simulink library "sm_suspension_templates_lib"  (R2021b)
settings: Solver=ode45  StartTime=0.0  StopTime=10.0  RelTol=1e-3  EnableMultiTasking=on
undefined symbols (not defined in the file or in its folder): dgrey, lbrown, lgrey, orange, rho_alum, X, Y, Z
libraries: sm_lib x133, $bdroot x10, nesl_utility x3, sm_double_wishbone_suspension_lib x2
(part 1 of 4)
settings Model: Creator=The MathWorks, Inc.  LastModifiedBy=The MathWorks, Inc.
settings SolverCC: AlgebraicLoopSolver=TrustRegion
settings DataIOCC: LimitDataPoints=on  SaveFormat=Array  ReturnWorkspaceOutputs=off
settings OptimizationCC: ExpressionDepthLimit=2147483647  LifeSpan=inf
settings DebuggingCC: UnderspecifiedInitializationDetection=Classic  MergeDetectMultiDrivingBlocksExec=none  SolverPrmCheckMsg=warning  AllowSymbolicDim=off  StateNameClashWarn=warning  SFUnexpectedBacktrackingDiag=warning  SFNoUnconditionalDefaultTransitionDiag=warning  SFExecutionAtInitializationDiag=none  SFMachineParentedDataDiag=warning  ArithmeticOperatorsInVariantConditions=warning
settings HardwareCC: ProdBitPerPointer=32  ProdBitPerSizeT=32  ProdBitPerPtrDiffT=32  ProdLargestAtomicFloat=None  ProdIntDivRoundTo=Undefined  ProdEndianess=Unspecified  ProdWordSize=32  ProdHWDeviceType=32-bit Generic
settings ModelReferenceCC: PropagateSignalLabelsOutOfModel=off
settings SFSimCC: SimUseLocalCustomCode=off  CustomCodeUndefinedFunction=UseInterfaceOnly
settings RTWCC: RTWUseLocalCustomCode=off
settings CodeAppCC: StateflowObjectComments=on
settings GRTTargetCC: TargetLangStandard=C89/C90 (ANSI)
settings ConfigComp: CovMetricSettings=dw  CovSaveCumulativeToWorkspaceVar=on  CovSaveSingleToWorkspaceVar=on  CovExternalEMLEnable=off  CovSFcnEnable=off

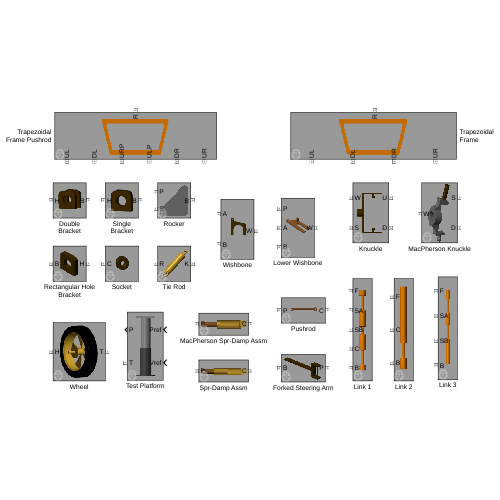
[thumbnail: Simulink's stored preview of the top-level diagram]
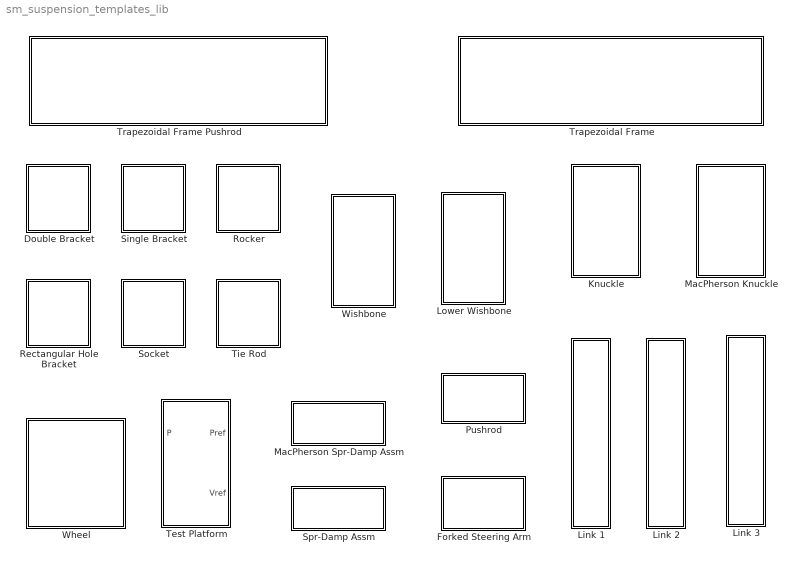
== system sm_suspension_templates_lib ==
  Double Bracket : Subsystem  mask(Bracket){L=4, W=4, T=1, S=1.5, Rh=1, rho=2700, clr=[0.3 0.2 0]}
      mask prompts: L "Length (cm):"; W "Width (cm):"; T "Thickness (cm):"; S "Spacing (cm):"; Rh "Hole radius (cm):"; rho "Density (kg/m^3):"; clr "Color ([r g b]):"
      mask help: This block models a rectangular bracket with two flanges. The port B corresponds to the base of the bracket and the port H corresponds to the bracket hole.
      mask init:
      | bracket_xsec = [W/2 -L/2; W/2 L/2; -W/2 L/2; -W/2 -L/2];
      | bracket_xsec = simmechanics.demohelpers.round_corners(bracket_xsec,[2 3],1,5);
      | 
      | theta = linspace(3*pi/2,-pi/2,100)';
      | bracket_xsec = [bracket_xsec; bracket_xsec(1,:);
      |                 Rh*cos(theta) Rh*sin(theta)];
      mask DialogControl ParameterTabVar0 Prompt: Dimensions
      mask DialogControl ParameterTabVar01 Prompt: Material Properties
      mask Display:
      | image(imread(fullfile(matlabroot,...
      |     'toolbox','physmod','sm','smdemos',...
      |     'suspension_templates','images','sm_isuspension_dbracket.png')));
      | 
      | port_label('LConn',1,'H');
      | port_label('RConn',1,'B');
  Forked Steering Arm : Subsystem  mask(Forked Steering Arm){L=20, W=2, Lf=4, Hf=10, Of=0, T=1, Rp=0.25, Rr=0.25, rho=2700, clr=[0.3 0.2 0]}
      mask prompts: L "Length of link (cm):"; W "Width of link (cm):"; Lf "Length of forked section (cm):"; Hf "Height of forked section (cm):"; Of "Offset of forked section (cm):"; T "Thickness of link (cm):"; Rp "Pin radius (cm):"; Rr "Chamfer/fillet radius (cm):"; rho "Density (kg/m^3)"; clr "Color ([r g b]):"
      mask help: This block models a steering arm that rigidly connects to the steering knuckle and is pushed/pulled by the tie rod to steer the vehicle. The port B corresponds to the attachment point of the arm to the knuckle and the port P refers to the pin frame where the arm attaches to the tie rod.
      mask init:
      | fork_xsec = [ -(L-Lf+T/2) -T/2; 
      |               -T/2 -T/2; 
      |               -T/2 -Hf/2+Of;
      |               Lf-T/2 -Hf/2+Of; 
      |               Lf-T/2 -(Hf/2-T)+Of; 
      |               T/2 -(Hf/2-T)+Of;
      |               T/2 (Hf/2-T)+Of; 
      |               Lf-T/2 (Hf/2-T)+Of; 
      |               Lf-T/2 Hf/2+Of;
      |               -T/2 Hf/2+Of;  
      |               -T/2 T/2; 
      |               -(L-Lf+T/2) T/2];
      | 
      | fork_xsec = simmechanics.demohelpers.round_corners(fork_xsec,2:11,Rr,5);
      mask DialogControl ParameterTabVar0 Prompt: Dimensions
      mask DialogControl ParameterTabVar01 Prompt: Material Properties
      mask Display:
      | image(fullfile(matlabroot,'toolbox','physmod','sm','smdemos','suspension_templates','images','sm_isuspension_steerarm.png'));
      | port_label('LConn',1,'B');
      | port_label('RConn',1,'P');
  Knuckle : Subsystem  mask(Steering knuckle){H=43, L=8, T=1, Wpr=2.5, Hpr=8, Wc=10, Rd=2, Hd=6, Rr=0.3, Rt=2, Rb=1, Rp=0.5, Hp=3, Ls=20, Ws=2, Ts=1, Hsf=10, Lsf=4, Osf=0, Rsp=0.5, Rsr=0.25, Rev=off, rho=2700, clr=[0.5 0.5 0.5]}
      mask prompts: H "Height (cm):"; L "Length (cm):"; T "Thickness (cm):"; Wpr "Width of wheel attach projection (cm):"; Hpr "Height of wheel attach projection (cm):"; Wc "Width of wishbone connectors (cm):"; Rd "Drive shaft hole radius (cm):"; Hd "Drive shaft bearing housing height (cm):"; Rr "Chamfer/fillet radius (cm):"; Rt "Transition radius to wheel attach projection (cm):"; Rb "Ball radius (cm):"; Rp "Pin radius (cm):"; Hp "Pin height (cm):"; Ls "Length of arm (cm):"; Ws "Width of arm (cm):"; Ts "Thickness of arm (cm):"; Hsf "Height of forked section (cm):"; Lsf "Length of forked section (cm):"; Osf "Offset of forked section (cm):"; Rsp "Pin radius (cm):"; Rsr "Chamfer/fillet radius (cm):"; Rev "Reverse direction:"; rho "Density (kg/m^3):"; clr "Color ([r g b]):"
      mask help: This block models a steering knuckle. The wheel hub attaches to the steering knuckle. The steering knuckle attaches to the wishbone links. The ports U and D correspond to the frames where the knuckle connects to the wishbone links. The port W corresponds to the frame where the wheel hub attaches to the knuckle. The knuckle also has a rigidly attached steering arm that attaches to the steering rack via tie rods. The port S corresponds to the frame where the steering arm attaches to the tie rod.
      mask init:
      | s_knuckle_xsec = [0 -Hd/2; 0 -Hpr/2; Wpr -Hpr/2; Wpr -H/2;
      |                 Wpr+Wc -H/2; Wpr+Wc -H/2+T; Wpr+T -H/2+T;
      |                  Wpr+T -Hd/2];
      | 
      | s_knuckle_xsec = simmechanics.demohelpers.round_corners(s_knuckle_xsec, 2:7, ...
      |                              [Rr Rt Rr*ones(1,4)], 20);
      | 
      | n_knuckle_xsec = flipud([s_knuckle_xsec(:,1) -s_knuckle_xsec(:,2)]);                         
      | 
      | Roh = sqrt((L/2)^2 + (Hd/2)^2);
      | phi = atan2(Hd,L);
      | theta = linspace(pi/2-phi,pi/2+phi,50)';
      | sh_xsec = [Roh*cos(theta) Roh*sin(theta)];
      | theta = linspace(3*pi/2-phi,3*pi/2+phi,50)';
      | sh_xsec = [sh_xsec; Roh*cos(theta) Roh*sin(theta)];
      | theta = linspace(5*pi/2-phi,pi/2-phi,100)';
      | sh_xsec = [sh_xsec; sh_xsec(1,:); Rd*cos(theta) Rd*sin(theta)];
      | 
      | % Convert Rev variable into +/- 1 instead of 0 or 1
      | sgn = (2*Rev-1);
      mask DialogControl ParameterTabVar0 Prompt: Dimensions
      mask DialogControl ParameterTabVar01 Prompt: Ball
      mask DialogControl ParameterTabVar012 Prompt: Steer Arm
      mask DialogControl ParameterTabVar0123 Prompt: Material Properties
      mask Display:
      | image(fullfile(matlabroot,'toolbox','physmod','sm','smdemos','suspension_templates','images','sm_isuspension_knuckle.png'));
      | port_label('RConn',1,'U');
      | port_label('RConn',2,'D');
      | port_label('LConn',1,'W');
      | port_label('LConn',2,'S');
  Link 1 : Subsystem  mask(Link 1){L=30, Ro=3, Ri=2, Lw=4, Ls=3, Ld=18, Ow=0, Rr=0.1, rho=2700, clr=[0.5 0.5 0.5]}
      mask prompts: L "Length of link (cm):"; Ro "Outer radius of link (cm):"; Ri "Inner radius of link (cm):"; Lw "Length of wishbone arm hinge slot (cm):"; Ls "Length of spring damper hinge slot (cm):"; Ld "Separation between wishbone arms (cm):"; Ow "Wishbone arms offset (cm):"; Rr "Chamfer/fillet radius (cm):"; rho "Density (kg/m^3):"; clr "Color ([r g b]):"
      mask help: This block models a cylindrical link that connects the trapezoidal frames and carries the wishbone links and the spring damper. The ports B and F correspond to the points at which the link attaches rigidly to the trapeziodal frames. The ports SA and SB correspond to the points at which the wish bone link arms attach. The port C correspond to the point at which the spring-damper assembly attaches.
      mask init:
      | link_xsec = [0 -L/2; Ro -L/2; ...
      |              Ro -Ld/2-Lw/2+Ow; Ri -Ld/2-Lw/2+Ow; ...
      |              Ri -Ld/2+Lw/2+Ow; Ro -Ld/2+Lw/2+Ow; ...
      |              Ro -Ls/2+Ow; Ri -Ls/2+Ow; ...
      |              Ri Ls/2+Ow; Ro Ls/2+Ow; ...
      |              Ro Ld/2-Lw/2+Ow; Ri Ld/2-Lw/2+Ow; ...
      |              Ri Ld/2+Lw/2+Ow; Ro Ld/2+Lw/2+Ow; ...
      |              Ro L/2; 0 L/2];
      | link_xsec = simmechanics.demohelpers.round_corners(link_xsec,[3:14],Rr,10);
      mask DialogControl ParameterTabVar0 Prompt: Dimensions
      mask DialogControl ParameterTabVar01 Prompt: Material Properties
      mask Display:
      | image(imread(fullfile(matlabroot,...
      |     'toolbox','physmod','sm','smdemos',...
      |     'suspension_templates','images','sm_isuspension_link1.png')));
      | 
      | port_label('LConn',1,'F');
      | port_label('LConn',2,'SA');
      | port_label('LConn',3,'SB');
      | port_label('LConn',4,'C');
      | port_label('LConn',5,'B');
  Link 2 : Subsystem  mask(Link 2){L=30, Ro=1.5, Ri=0.75, Ls=3, Ow=0, Rr=0.2, rho=2700, clr=[255 140 0]/255}
      mask prompts: L "Length of link (cm):"; Ro "Outer radius of link (cm):"; Ri "Inner radius of link (cm):"; Ls "Length of spring damper hinge slot (cm):"; Ow "Spring damper offset (cm):"; Rr "Chamfer/fillet radius (cm):"; rho "Density (kg/m^3):"; clr "Color ([r g b]:"
      mask help: This block models a cylindrical link that connects the trapezoidal frames and carries the wishbone links and the spring damper. The ports B and F correspond to the points at which the link attaches rigidly to the trapeziodal frames. The port C correspond to the point at which the spring-damper assembly attaches.
      mask init:
      | link_xsec = [0  -L/2;...
      |              Ro -L/2; ...
      |              Ro  Ow - Ls/2; ...
      |              Ri  Ow - Ls/2; ...
      |              Ri  Ow + Ls/2; ...
      |              Ro  Ow + Ls/2; ...
      |              Ro  L/2; ...
      |              0   L/2];
      | link_xsec = simmechanics.demohelpers.round_corners(link_xsec,[4:7],Rr,10);
      mask DialogControl ParameterTabVar0 Prompt: Dimensions
      mask DialogControl ParameterTabVar01 Prompt: Material Properties
      mask Display:
      | image(imread(fullfile(matlabroot,...
      |     'toolbox','physmod','sm','smdemos',...
      |     'suspension_templates','images','sm_isuspension_link2.png')));
      | 
      | port_label('LConn',1,'F');
      | port_label('LConn',2,'C');
      | port_label('LConn',3,'B');
  Link 3 : Subsystem  mask(Link 3){L=30, Ro=1.5, Ri=0.75, Lw=5.5, Ld=10.25, Ow=3.125, Rr=0.2, rho=2700, clr=[255 140 0]/255}
      mask prompts: L "Length of link (cm):"; Ro "Outer radius of link (cm):"; Ri "Inner radius of link (cm):"; Lw "Length of wishbone arm hinge slot (cm):"; Ld "Separation between wishbone arms (cm):"; Ow "Wishbone arms offset (cm):"; Rr "Chamfer/fillet radius (cm):"; rho "Density (kg/m^3):"; clr "Color ([r g b]:"
      mask help: This block models a cylindrical link that connects the trapezoidal frames and carries the wishbone links and the spring damper. The ports B and F correspond to the points at which the link attaches rigidly to the trapeziodal frames. The ports SA and SB correspond to the points at which the wish bone link arms attach.
      mask init:
      | link_xsec = [0  -L/2; ...
      |              Ro -L/2; ...
      |              Ro -Ld/2-Lw/2+Ow; ...
      |              Ri -Ld/2-Lw/2+Ow; ...
      |              Ri -Ld/2+Lw/2+Ow; ...
      |              Ro -Ld/2+Lw/2+Ow; ...
      |              Ro  Ld/2-Lw/2+Ow; ...
      |              Ri  Ld/2-Lw/2+Ow; ...
      |              Ri  Ld/2+Lw/2+Ow; ...
      |              Ro  Ld/2+Lw/2+Ow; ...
      |              Ro  L/2; ...
      |              0   L/2];
      | link_xsec = simmechanics.demohelpers.round_corners(link_xsec,[3:8],Rr,10);
      mask DialogControl ParameterTabVar0 Prompt: Dimensions
      mask DialogControl ParameterTabVar01 Prompt: Material Properties
      mask Display:
      | image(imread(fullfile(matlabroot,...
      |     'toolbox','physmod','sm','smdemos',...
      |     'suspension_templates','images','sm_isuspension_link3.png')));
      | 
      | port_label('LConn',1,'F');
      | port_label('LConn',2,'SA');
      | port_label('LConn',3,'SB');
      | port_label('LConn',4,'B');
  Lower Wishbone : Subsystem  mask(Lower Wishbone){L1=36, L2=25, L3=5, W3=5, W=14.75, T=2, Rb=2.875, Ob=15, Rev=off, Lb=4, Rsh=0.75, Rs=2, Hi=1.4, Rh=1, Oh=3.0625, Odb=10, Wdb=4, Ldb=4, Tdb=1, Sdb=1.5, Rhdb=1, rho=rho_alum, clr=lbrown}
      mask prompts: L1 "Long side length (cm):"; L2 "Short side length (cm):"; L3 "Wheel link length (cm):"; W3 "Width of wheel link (cm):"; W "Width of entire link (cm):"; T "Thickness (cm):"; Rb "Radius of base (cm):"; Ob "Base arc offset (cm):"; Rev "Reverse bracket and socket axes"; Lb "Supporting bracket length (cm):"; Rsh "Supporting bracket hole radius (cm):"; Rs "Wheel hub socket radius (cm):"; Hi "Wheel hub inner height (cm):"; Rh "Wheel hub hole radius (cm):"; Oh "Wheel hub hole offset (cm):"; Odb "Offset (cm):"; Wdb "Width (cm):"; Ldb "Length (cm):"; Tdb "Thickness (cm):"; Sdb "Spacing (cm):"; Rhdb "Hole radius (cm):"; rho "Density (kg/m^3):"; clr "Color ([r g b]:"
      mask help: This block models a wishbone link. The wishbone links are attached to the frame and they carry the wheel assembly. The ports A and B correspond to the frames at the hinge points where the wishbone link attaches to the chassis. Port P corresponds to the attachment frame for a Spring-Damper assembly in a double wishbone configuration and the pushrod linkage attachment in a pushrod configuration. Port W corresponds to the point where the wishbone link attaches to the steering knuckle.
      mask init:
      | wishbone_xsec = [Rb 0; W/2 0; W/2 L1; W/2-W3 L1; 
      |                  W/2-W3 L1-L3; -W/2 L2; -W/2 0; -Rb 0];
      | 
      | theta = linspace(pi,0,100)';
      | wishbone_xsec = [wishbone_xsec; Rb*cos(theta) Rb*sin(theta)+Ob];
      | 
      | wishbone_xsec = simmechanics.demohelpers.round_corners(wishbone_xsec, ...
      |                               [3 4 5 6], ...
      |                               [1 1 1 3], ...
      |                               5);
      | 
      | theta = linspace(3*pi/2,-pi/2,100)';
      | wishbone_xsec = [wishbone_xsec; 
      |                  wishbone_xsec(1,:);
      |                  W/2-W3/2+Rh*cos(theta) Rh*sin(theta)+L1-Oh];
      | 
      | bracket_xsec = [T/2 0; T/2 Lb; -T/2 Lb; -T/2 0];
      | bracket_xsec = simmechanics.demohelpers.round_corners(bracket_xsec,[2 3],1,5);
      | bracket_xsec = [bracket_xsec; 
      |                 bracket_xsec(1,:);
      |                 Rsh*cos(theta) Rsh*sin(theta)+Lb/2];
      |             
      | sgn = 2*Rev-1;
      settings: CloseFcn=disp('close')
      mask Callback Rev: set_param([gcb '/Wish Bone'],'Rev',get_param(gcbh,'Rev'));
      mask DialogControl ParameterTabVar0 Prompt: Wishbone
      mask DialogControl ParameterTabVar01 Prompt: Brackets
      mask DialogControl ParameterTabVar012 Prompt: Socket
      mask DialogControl ParameterTabVar0123 Prompt: Damper Bracket
      mask DialogControl ParameterTabVar01234 Prompt: Material Properties
      mask Display:
      | image(imread(fullfile(matlabroot,...
      |     'toolbox','physmod','sm','smdemos',...
      |     'suspension_templates','images','sm_isuspension_lowerwbone.png')));
      | 
      | port_label('LConn',1,'P');
      | port_label('LConn',2,'A');
      | port_label('LConn',3,'B');
      | port_label('RConn',1,'W');
  MacPherson Knuckle : Subsystem  mask(MacPherson Knuckle){SD_theta=30, Rb=1, Hub_L=15, Rev=off, rho=2700, clr=[0.5 0.5 0.5]}
      mask prompts: SD_theta "Spring-Damper Angle (deg):"; Rb "Ball Diameter (cm):"; Hub_L "Hub Length (cm):"; Rev "Reverse"; rho "Density (kg/m^3):"; clr "Color ([r g b]):"
      mask help: This block provides a steering knuckle for the MacPherson suspension. The knuckle attaches to the wheel hub, damper assembly and lower suspension wishbone. Port S corresponds to the frame were the spring-damper assembly is attached. Port D corresponds to the frame were the lower wish bone link is attached, and port W corresponds to the frame were the wheel hub is attached.
      mask init:
      | rho = 2700;
      | clr = [0.5 0.5 0.5];
      | T = 1;
      | Wc = 5;
      | H = Hub_L;
      | Wpr = 2.5;
      | L = 3;
      | Hpr = 8;
      | T = 1;
      | Wpr = 2.5;
      | Rd = 2;
      | Hd = 6;
      | Hp = 2;
      | Rp = 0.5;
      | Rb = 1;
      | Rr = 0.3;
      | Rt = 2;
      | 
      | angle = SD_theta*pi/180;
      | hh = sin(angle)*Wc/2;
      | s_knuckle_xsec = [0 -Hd/2; 0 -Hpr/2; Wpr -Hpr/2; Wpr -H/2;
      |                 Wpr+Wc -H/2; Wpr+Wc -H/2+T; Wpr+T -H/2+T;
      |                  Wpr+T -Hd/2];
      | hh = [0 0 0 0 hh hh hh 0]';
      | n_knuckle_xsec = [s_knuckle_xsec(:,1) s_knuckle_xsec(:,2)+hh];
      | s_knuckle_xsec = simmechanics.demohelpers.round_corners(s_knuckle_xsec, 2:7, ...
      |                              [Rr Rt Rr*ones(1,4)], 20);  
      | n_knuckle_xsec = simmechanics.demohelpers.round_corners(n_knuckle_xsec, 2:7, ...
      |                              [Rr Rt Rr*ones(1,4)], 20); 
      | n_knuckle_xsec = flipud([n_knuckle_xsec(:,1) -n_knuckle_xsec(:,2)]);
      | 
      | Roh = sqrt((L/2)^2 + (Hd/2)^2);
      | phi = atan2(Hd,L);
      | theta = linspace(pi/2-phi,pi/2+phi,50)';
      | sh_xsec = [Roh*cos(theta) Roh*sin(theta)];
      | theta = linspace(3*pi/2-phi,3*pi/2+phi,50)';
      | sh_xsec = [sh_xsec; Roh*cos(theta) Roh*sin(theta)];
      | theta = linspace(5*pi/2-phi,pi/2-phi,100)';
      | sh_xsec = [sh_xsec; sh_xsec(1,:); Rd*cos(theta) Rd*sin(theta)];
      mask DialogControl Container3 Prompt: Dimensions
      mask DialogControl Container6 Prompt: Material Properties
      mask Display:
      | image(fullfile(matlabroot,'toolbox','physmod','sm','smdemos','suspension_templates','images','sm_isuspension_macphersonknuckle.png'));
      | port_label('RConn',1,'S');
      | port_label('RConn',2,'D');
      | port_label('LConn',1,'W');
  MacPherson Spr-Damp Assm : Subsystem  mask(MacPherson Spring-Damper){Ks=2000, Kb=1500, Ls=15, Lc=22, Rci=2, Rco=3, Lp=15, Rr=0.3, Lb=4, Wb=4, Tb=1, Rbh=0.75, rho=2700, cclr=[0.9 0.7 0.2], pclr=[0.55    0.35   0.17]}
      mask prompts: Ks "Spring constant (N/m):"; Kb "Damping coefficient (Ns/m)"; Ls "Spring natural length (cm):"; Lc "Length of cylinder (cm):"; Rci "Inner radius of cylinder (cm):"; Rco "Outer radius of cylinder (cm):"; Lp "Length of piston (cm):"; Rr "Chamfer/fillet radius (cm):"; Lb "Length (cm):"; Wb "Width (cm):"; Tb "Thickness (cm):"; Rbh "Hole radius (cm):"; rho "Density (kg/m^3):"; cclr "Cylinder color ([r g b]):"; pclr "Piston color ([r g b]):"
      mask help: This block models a spring-damper system for a MacPherson style steering knuckle. The port C corresponds to the bracket on the cylinder and the port P corresponds to the furthest point in the piston.
      mask init:
      | dr = Rco-Rci;
      | cyl_xsec = [0 -Lc/2; Rco -Lc/2; 
      |             Rco Lc/2; Rci Lc/2; 
      |             Rci -Lc/2+dr; 0 -Lc/2+dr];
      | cyl_xsec = simmechanics.demohelpers.round_corners(cyl_xsec,2:5,Rr,10);
      | 
      | piston_xsec = [0 -Lp/2; Rci -Lp/2; Rci Lp/2; 0 Lp/2];
      | piston_xsec = simmechanics.demohelpers.round_corners(piston_xsec,2:3,Rr,10);
      mask DialogControl ParameterTabVar0 Prompt: Spring/Damper
      mask DialogControl ParameterTabVar01 Prompt: Dimensions
      mask DialogControl ParameterTabVar012 Prompt: Brackets
      mask DialogControl ParameterTabVar0123 Prompt: Material Properties
      mask Display:
      | image(fullfile(matlabroot,'toolbox','physmod','sm','smdemos','suspension_templates','images','sm_isuspension_macphersonsprdamp.png'));port_label('LConn',1,'C');
      | port_label('RConn',1,'P');
  Pushrod : Subsystem  mask(Pushrod){Rci=1, Lp=22, Lb=4, Wb=4, Tb=1, Rbh=0.75, rho=2700, cclr=[0.9 0.7 0.2], pclr=[0.55    0.35   0.17]}
      mask prompts: Rci "Radius of Rod (cm):"; Lp "Length of Rod (cm):"; Lb "Length (cm):"; Wb "Width (cm):"; Tb "Thickness (cm):"; Rbh "Hole radius (cm):"; rho "Density (kg/m^3):"; cclr "Cylinder color ([r g b]):"; pclr "Piston color ([r g b]):"
      mask help: This block models a solid linkage with two brackets that can be used as a pushrod. Ports C and P correspond to the frames at the center of the two brackets located in the ends of the linkage.
      mask init:
      | % dr = Rco-Rci;
      | % cyl_xsec = [0 -Lc/2; Rco -Lc/2; 
      | %             Rco Lc/2; Rci Lc/2; 
      | %             Rci -Lc/2+dr; 0 -Lc/2+dr];
      | % cyl_xsec = simmechanics.demohelpers.round_corners(cyl_xsec,2:5,Rr,10);
      | 
      | piston_xsec = [0 -Lp/2; Rci -Lp/2; Rci Lp/2; 0 Lp/2];
      | %piston_xsec = simmechanics.demohelpers.round_corners(piston_xsec,2:3,Rr,10);
      mask DialogControl ParameterTabVar01 Prompt: Dimensions
      mask DialogControl ParameterTabVar012 Prompt: Brackets
      mask DialogControl ParameterTabVar0123 Prompt: Material Properties
      mask Display:
      | image(imread(fullfile(matlabroot,...
      |     'toolbox','physmod','sm','smdemos',...
      |     'suspension_templates','images','sm_isuspension_rod.png')));
      | 
      | port_label('LConn',1,'C');
      | port_label('RConn',1,'P');
  Rectangular Hole Bracket : Subsystem  mask(Bracket){L=4, W=4, T=1, Lh=2, Wh=2, Rr=0.5, rho=2700, clr=[0.3 0.2 0.0]}
      mask prompts: L "Length (cm):"; W "Width (cm):"; T "Thickness (cm):"; Lh "Hole length (cm):"; Wh "Hole width (cm):"; Rr "Chamfer/fillet radius (cm):"; rho "Density (kg/m^3):"; clr "Color ([r g b]):"
      mask help: This block models a rectangular bracket with a rounded rectangular hole. The port B corresponds to the base of the bracket and the port H corresponds to the bracket hole.
      mask init:
      | bracket_xsec = [W/2 -L/2; W/2 L/2; -W/2 L/2; 
      |                 -W/2 -L/2; W/2 -L/2];
      | bracket_xsec = simmechanics.demohelpers.round_corners(bracket_xsec,[2 3],Rr,5);
      | 
      | hole_xsec = [Wh/2 -Lh/2; -Wh/2 -Lh/2; -Wh/2 Lh/2; 
      |              Wh/2 Lh/2];
      | hole_xsec = simmechanics.demohelpers.round_corners(hole_xsec,1:4,Rr,5);         
      |          
      | bracket_xsec = [bracket_xsec; 
      |                 hole_xsec; hole_xsec(1,:)];
      mask DialogControl ParameterTabVar0 Prompt: Dimensions
      mask DialogControl ParameterTabVar01 Prompt: Material Properties
      mask Display:
      | image(imread(fullfile(matlabroot,...
      |     'toolbox','physmod','sm','smdemos',...
      |     'suspension_templates','images','sm_isuspension_sqbracket.png')));
      | 
      | port_label('LConn',1,'B');
      | port_label('RConn',1,'H');
  Rocker : Subsystem  mask(Rocker){InputArmLength=10, Ratio=1, Thickness=3, Rev=off, rho=8050, rgb=[0.5 0.5 0.5]}
      mask prompts: InputArmLength "Input arm length (cm):"; Ratio "Motion ratio (input/output):"; Thickness "Thickness (cm):"; Rev "Reverse base frame axes"; rho "Density (kg/m^3):"; rgb "Color ([r g b]):"
      mask help: This block models a rocker that translates the motion provided by a pushrod connected to a wishbone link into a rotary force. The rocker provides a variable motion ratio between the input (pushrod) and the output (spring-damper assembly) of the rotating linkage. Port S corresponds to the frame of a spring-damper assembly in a pushrod/pullrod suspension, and port P corresponds to the frame of the pushrod/pullrod. Port B corresponds to the base frame associated as the rotating point of the linkage.
      mask init:
      | alpha=atan(Ratio);
      | beta=(pi/2-alpha);
      | Rh=1;
      | Ra=1.6;
      | theta = linspace(3*pi/2,-pi/2,100)';
      | theta1= linspace(3*pi/4,2*pi,100)';
      | theta2= linspace(0,3*pi/4,100)';
      | theta3= linspace(pi,2*pi,100)';
      | theta4= linspace(0,pi,100)';
      | thetaBL=linspace(pi,3*pi/2,10)';
      | thetaBR1=linspace(3*pi/2,2*pi,7)';
      | thetaBR2=linspace(0,alpha,4)';
      | thetaTL=linspace(pi/2-beta,pi,10)';
      | Rocker_xsec=[(Ra*Rh)*cos(thetaBL),(Ra*Rh)*sin(thetaBL);
      |     InputArmLength*Ratio+(Ra*Rh)*cos(thetaBR1),(Ra*Rh)*sin(thetaBR1);
      |     InputArmLength*Ratio+(Ra*Rh)*cos(thetaBR2),(Ra*Rh)*sin(thetaBR2);
      |    (Ra*Rh)*cos(thetaTL),InputArmLength+(Ra*Rh)*sin(thetaTL)];
      | sgn=2*Rev-1;
      mask DialogControl Container4 Prompt: Dimensions
      mask DialogControl Container8 Prompt: Material Properties
      mask Display:
      | image(imread(fullfile(matlabroot,...
      |     'toolbox','physmod','sm','smdemos',...
      |     'suspension_templates','images','sm_isuspension_rocker.png')));
      | 
      | port_label('LConn',1,'P');
      | port_label('LConn',2,'S');
      | port_label('RConn',1,'B');
  Single Bracket : Subsystem  mask(Bracket){L=4, W=4, T=1, Rh=1, rho=2700, clr=[0.5 0.5 0.5]}
      mask prompts: L "Length (cm):"; W "Width (cm):"; T "Thickness (cm):"; Rh "Hole radius (cm):"; rho "Density (kg/m^3):"; clr "Color ([r g b]):"
      mask help: This block models a rectangular bracket with a circular hole. The port B corresponds to the base of the bracket and the port H corresponds to the bracket hole.
      mask init: same as sm_suspension_templates_lib/Double Bracket
      mask DialogControl ParameterTabVar0 Prompt: Dimensions
      mask DialogControl ParameterTabVar01 Prompt: Material Properties
      mask Display:
      | image(imread(fullfile(matlabroot,...
      |     'toolbox','physmod','sm','smdemos',...
      |     'suspension_templates','images','sm_isuspension_sbracket.png')));
      | 
      | port_label('LConn',1,'H');
      | port_label('RConn',1,'B');
  Socket : Subsystem  mask(Socket){Ro=2, Ri=1, Ho=1.5, Hi=1.4, Rr=0.2, rho=2700, clr=[0.3 0.2 0.0]}
      mask prompts: Ro "Outer radius of socket (cm):"; Ri "Ball radius (cm):"; Ho "Outer height of socket (cm):"; Hi "Height of inner curved surface (cm):"; Rr "Chamfer/fillet radius (cm):"; rho "Density (kg/m^3):"; clr "Color ([r g b]):"
      mask help: This block models a socket that can hold a ball. The port C refers to the center of the socket.
      mask init:
      | phi = asin(Hi/(2*Ri));
      | theta = linspace(phi,-phi,25)';
      | 
      | socket_xsec = [Ri -Ho/2; Ro -Ho/2; Ro Ho/2; Ri Ho/2;
      |                Ri*cos(theta) Ri*sin(theta)];
      mask DialogControl ParameterTabVar0 Prompt: Dimensions
      mask DialogControl ParameterTabVar01 Prompt: Material Properties
      mask Display:
      | image(imread(fullfile(matlabroot,...
      |     'toolbox','physmod','sm','smdemos',...
      |     'suspension_templates','images','sm_isuspension_socket.png')));
      | 
      | port_label('LConn',1,'C');
  Spr-Damp Assm : Subsystem  mask(Spring-Damper){Ks=2000, Kb=1500, Ls=15, Lc=22, Rci=2, Rco=3, Lp=17, Rr=0.3, Lb=4, Wb=4, Tb=1, Rbh=0.75, rho=2700, cclr=[0.9 0.7 0.2], pclr=[0.55    0.35   0.17]}
      mask prompts: Ks "Spring constant (N/m):"; Kb "Damping coefficient (Ns/m)"; Ls "Spring natural length (cm):"; Lc "Length of cylinder (cm):"; Rci "Inner radius of cylinder (cm):"; Rco "Outer radius of cylinder (cm):"; Lp "Length of piston (cm):"; Rr "Chamfer/fillet radius (cm):"; Lb "Length (cm):"; Wb "Width (cm):"; Tb "Thickness (cm):"; Rbh "Hole radius (cm):"; rho "Density (kg/m^3):"; cclr "Cylinder color ([r g b]):"; pclr "Piston color ([r g b]):"
      mask help: This block models a spring-damper system. The port C corresponds to the bracket on the cylinder and the port P corresponds to the bracket on the piston side.
      mask init: same as sm_suspension_templates_lib/MacPherson Spr-Damp Assm
      mask DialogControl ParameterTabVar0 Prompt: Spring/Damper
      mask DialogControl ParameterTabVar01 Prompt: Dimensions
      mask DialogControl ParameterTabVar012 Prompt: Brackets
      mask DialogControl ParameterTabVar0123 Prompt: Material Properties
      mask Display:
      | image(fullfile(matlabroot,'toolbox','physmod','sm','smdemos','suspension_templates','images','sm_isuspension_sprdampassm.png'));
      | port_label('LConn',1,'C');
      | port_label('RConn',1,'P');
  Test Platform : Subsystem  mask(Suspension Test Platform){Ro=12, Ri=10, Rf=20, Tf=2, Hc=40, cclr=dgrey, loc=[80 -25 0], Rip=8, Hp=60, pclr=lgrey, L=40, W=40, H=3, clr=lgrey, Kp=1e4, Kd=100, rho=rho_alum}
      mask prompts: Ro "Hoist cylinder outer radius (cm):"; Ri "Hoist cylinder inner radius (cm):"; Rf "Hoist cylinder flange radius (cm):"; Tf "Hoist cylinder flange thickness (cm):"; Hc "Hoist cylinder height (cm):"; cclr "Cylinder color ([r g b]):"; loc "Location of hoist ([x y z]) (cm):"; Rip "Hoist piston inner radius (cm):"; Hp "Hoist piston height (cm):"; pclr "Piston color ([r g b]):"; L "Platform length (cm):"; W "Platform width (cm):"; H "Platform thickness (cm):"; clr "Color ([r g b]):"; Kp "Proportional Gain"; Kd "Derivative Gain"; rho "Density (kg/m^3):"
      mask help: This block models a testing platform that moves the tires up and down (imitating road profile). The testing platform has a PD controller that tracks the reference road profile based on the desired profile height (Pref) and velocity (Vref). The output P is the actual platform height. The port T corresponds to the center of the top surface of the platform.
      mask init:
      | cyl_xsec = [Ri -Hc/2; Rf -Hc/2; Rf -Hc/2+Tf;
      |             Ro -Hc/2+Tf; Ro Hc/2; Ri Hc/2];
      |         
      | pist_xsec = [Rip -Hp/2; Ri -Hp/2; Ri Hp/2; Rip Hp/2];
      mask DialogControl ParameterTabVar0 Prompt: Cyl
      mask DialogControl ParameterTabVar01 Prompt: Piston
      mask DialogControl ParameterTabVar012 Prompt: Platform
      mask DialogControl ParameterTabVar0123 Prompt: Controller
      mask DialogControl ParameterTabVar01234 Prompt: Material Properties
      mask Display:
      | image(imread(fullfile(matlabroot,...
      |     'toolbox','physmod','sm','smdemos',...
      |     'suspension_templates','images','sm_isuspension_platform.png')));
      | 
      | port_label('input',1,'Pref');
      | port_label('input',2,'Vref');
      | port_label('RConn',1,'T');
      | port_label('output',1,'P');
  Tie Rod : Subsystem  mask(Tie Rod){L=20, R=2, Rr=0.5, Lb=3, Wb=2, Tb=0.5, Sb=1.5, Rs=0.5, Rb=0.5, Rh=0.3, rho=2700, tclr=[0.5 0.5 0.5], bclr=[0.5 0.5 0.5]}
      mask prompts: L "Length (cm):"; R "Radius (cm):"; Rr "Chamfer/fillet radius (cm):"; Lb "Length (cm):"; Wb "Width (cm):"; Tb "Thickness (cm):"; Sb "Spacing between flanges (cm):"; Rs "Socket radius (cm):"; Rb "Ball radius (cm):"; Rh "Hole radius (cm):"; rho "Density (kg/m^3):"; tclr "Tie rod color ([r g b]):"; bclr "Ball color ([r g b]):"
      mask help:
      | This block models a tie rod that connects the steering rack to the steering arm of the steering knuckle. The port K corresponds to the end connecting to the knuckle and the port R corresponds to the end connecting to the rack.
      | The tie rod has a ball-socket (spherical) joint at the steering arm end. The ball has a hole that attaches to the steering arm pin.
      mask init:
      | Lr = L/2 - Lb;
      | rod_xsec = [0 -Lr; R -Lr; R Lr; 0 Lr];
      | rod_xsec = simmechanics.demohelpers.round_corners(rod_xsec,2:3,Rr,5);
      | 
      | phi = acos(Rh/Rb);
      | theta = linspace(-phi,phi,25)';
      | ball_xsec = [Rb*cos(theta) Rb*sin(theta)];
      mask DialogControl ParameterTabVar0 Prompt: Rod
      mask DialogControl ParameterTabVar01 Prompt: Brackets
      mask DialogControl ParameterTabVar012 Prompt: Material Properties
      mask Display:
      | image(imread(fullfile(matlabroot,...
      |     'toolbox','physmod','sm','smdemos',...
      |     'suspension_templates','images','sm_isuspension_tierod.png')));
      | 
      | port_label('LConn',1,'R');
      | port_label('RConn',1,'K');
  Trapezoidal Frame : Subsystem  mask(Trapeziodal Frame){L1=80, L2=60, H=25, R=5, T=2, Tb=5, rho=2700, clr=[0.5 0.5 0.5]}
      mask prompts: L1 "Long side length of frame (cm):"; L2 "Short side length of frame (cm):"; H "Height of frame (cm):"; R "Radius of rounded corners (cm):"; T "Thickness of frame (cm):"; Tb "Thickness of frame bars (cm):"; rho "Density (kg/m^3):"; clr "Color ([r g b]):"
      mask help: This block models a trapeziodal frame that is part of the chassis on to which the suspension is mounted. The ports DR, DL, UR, UL correspond to the four corners of the frame. The port R corresponds to the central reference frame.
      mask init:
      | phi = atan2(H,(L1-L2)/2);
      | 
      | outer_xsec = [L2/2 -H/2; L1/2 H/2; -L1/2 H/2; -L2/2 -H/2];
      | 
      | inner_xsec = [ L2/2-Tb/tan((pi-phi)/2)    -(H/2-Tb);
      |                -L2/2+Tb/tan((pi-phi)/2)   -(H/2-Tb);
      |                -L1/2+Tb/tan(phi/2)          H/2-Tb;
      |                L1/2-Tb/tan(phi/2)           H/2-Tb];
      | 
      | % Frames are midway between the inner and outer 
      | % trapezium vertices           
      | frames = (outer_xsec+[inner_xsec(1,:); flipud(inner_xsec(2:end,:))])/2;
      | 
      | outer_xsec = simmechanics.demohelpers.round_corners(outer_xsec,[1 2 3 4],R,20);
      | inner_xsec = simmechanics.demohelpers.round_corners(inner_xsec,[1 2 3 4],R,20);       
      |           
      | frame_xsec = [outer_xsec; outer_xsec(1,:); ...
      |               inner_xsec; inner_xsec(1,:)];      
      |           
      | sec = frames(1,:);          
      | nec = frames(2,:);          
      | nwc = frames(3,:);          
      | swc = frames(4,:);
      mask DialogControl ParameterTabVar0 Prompt: Dimensions
      mask DialogControl ParameterTabVar01 Prompt: Material Properties
      mask Display:
      | image(imread(fullfile(matlabroot,...
      |     'toolbox','physmod','sm','smdemos',...
      |     'suspension_templates','images','sm_isuspension_frame.png')));
      | 
      | port_label('LConn',1,'UL');
      | port_label('LConn',2,'DL');
      | port_label('LConn',3,'DR');
      | port_label('LConn',4,'UR');
      | port_label('RConn',1,'R');
  Trapezoidal Frame Pushrod : Subsystem  mask(Trapeziodal Frame for Pushrod){PRstrut=40, L1=100, L2=75, H=40, R=2, T=2, Tb=5, rho=rho_alum, clr=orange}
      mask prompts: PRstrut "Pushrod support offset (cm):"; L1 "Long side length of frame (cm):"; L2 "Short side length of frame (cm):"; H "Height of frame (cm):"; R "Radius of rounded corners (cm):"; T "Thickness of frame (cm):"; Tb "Thickness of frame bars (cm):"; rho "Density (kg/m^3):"; clr "Color ([r g b]):"
      mask help: This block models a trapeziodal frame that is part of the chassis on to which the pushrod suspension is mounted. The ports DR, DL, UR, UL correspond to the four corners of the frame. The port R corresponds to the central reference frame. The port URP and ULP correspond to the mounting points of the damper supports.
      mask init:
      | phi = atan2(H,(L1-L2)/2);
      | 
      | outer_xsec = [L2/2 -H/2; L1/2 H/2; -L1/2 H/2; -L2/2 -H/2];
      | 
      | inner_xsec = [ L2/2-Tb/tan((pi-phi)/2)    -(H/2-Tb);
      |                -L2/2+Tb/tan((pi-phi)/2)   -(H/2-Tb);
      |                -L1/2+Tb/tan(phi/2)          H/2-Tb;
      |                L1/2-Tb/tan(phi/2)           H/2-Tb];
      | 
      | % Frames are midway between the inner and outer 
      | % trapezium vertices           
      | frames = (outer_xsec+[inner_xsec(1,:); flipud(inner_xsec(2:end,:))])/2;
      | 
      | outer_xsec = simmechanics.demohelpers.round_corners(outer_xsec,[1 2 3 4],R,20);
      | inner_xsec = simmechanics.demohelpers.round_corners(inner_xsec,[1 2 3 4],R,20);       
      |           
      | frame_xsec = [outer_xsec; outer_xsec(1,:); ...
      |               inner_xsec; inner_xsec(1,:)];      
      |           
      | sec = frames(1,:);      
      | nec = frames(2,:);          
      | nwc = frames(3,:);          
      | swc = frames(4,:);    
      | necp=[nec(1)-PRstrut nec(2)];
      | nwcp=[nwc(1)+PRstrut nwc(2)];
      mask DialogControl ParameterTabVar0 Prompt: Dimensions
      mask DialogControl ParameterTabVar01 Prompt: Material Properties
      mask Display:
      | image(imread(fullfile(matlabroot,...
      |     'toolbox','physmod','sm','smdemos',...
      |     'suspension_templates','images','sm_isuspension_frame.png')));
      | 
      | port_label('LConn',1,'UL');
      | port_label('LConn',2,'DL');
      | port_label('LConn',3,'URP');
      | port_label('LConn',4,'ULP');
      | port_label('LConn',5,'DR');
      | port_label('LConn',6,'UR');
      | port_label('RConn',1,'R');
  Wheel : Subsystem  mask(Wheel){Rti=25, Rto=30, Wt=15, Rtr=1, trho=1000, tclr=[0 0 0], Rhi=5, Rho=23, Ns=5, Ts=1, Wh=11, srho=2700, sclr=[0.5 0.5 0.5], Ls=6, Rs=2, Rb=10, Tb=1}
      mask prompts: Rti "Tire inner radius (cm):"; Rto "Tire outer radius (cm):"; Wt "Tire width (cm):"; Rtr "Chamfer/fillet radius (cm):"; trho "Density (kg/m^3):"; tclr "Color ([r  g b]):"; Rhi "Hub radius (cm):"; Rho "Outer radius of spokes (cm):"; Ns "Number of spokes:"; Ts "Thickness of spokes:"; Wh "Width of hub (cm):"; srho "Density (kg/m^3):"; sclr "Color ([r g b]):"; Ls "Shaft length (cm):"; Rs "Shaft radius (cm):"; Rb "Brake disc radius (cm):"; Tb "Brake disc thickness (cm):"
      mask help: This block models a wheel assembly. The port H corresponds to the center of the wheel hub. Port T corresponds to the bottom of the tire.
      mask init:
      | spk_angles = linspace(0,2*pi,Ns+1);
      | 
      | spokes_xsec = [];
      | r_indices = [];
      | wang = 20*pi/180;
      | for idx = 1:length(spk_angles)-1
      |     ang = spk_angles(idx);
      |     theta = linspace(ang-wang,ang+wang,20)';
      |     spokes_xsec = [spokes_xsec;
      |                    Rhi*cos(theta) Rhi*sin(theta)];
      |     theta = linspace(ang+wang, spk_angles(idx+1)-wang, 50)';
      |     len = length(spokes_xsec);
      |     r_indices = [r_indices len len+1];
      |     spokes_xsec = [spokes_xsec;
      |                    Rho*cos(theta) Rho*sin(theta)];
      | end
      | 
      | rim_xsec = [Rho -Wh/2; Rti -Wt/2; 
      |             Rti Wt/2; Rho Wh/2+Ts];
      | 
      | tire_xsec = [Rti -Wt/2; Rto -Wt/2; Rto Wt/2; Rti Wt/2];
      | tire_xsec = simmechanics.demohelpers.round_corners(tire_xsec,1:4,Rtr,10);
      mask DialogControl ParameterTabVar0 Prompt: Tire
      mask DialogControl ParameterTabVar01 Prompt: Hub
      mask DialogControl ParameterTabVar012 Prompt: Brake and Shaft
      mask Display:
      | image(imread(fullfile(matlabroot,...
      |     'toolbox','physmod','sm','smdemos',...
      |     'suspension_templates','images','sm_isuspension_wheel.png')));
      | 
      | port_label('LConn',1,'H');
      | port_label('RConn',1,'T');
  Wishbone : Subsystem  mask(Wishbone){L1=25, L2=15, L3=5, W3=5, W=25, T=3, Rb=8, Ob=5, Rev=off, Lb=4, Rsh=1, Rs=2, Hi=1.4, Rh=1, Oh=3, rho=2700, clr=[0.5 0.5 0.5]}
      mask prompts: L1 "Long side length (cm):"; L2 "Short side length (cm):"; L3 "Wheel link length (cm):"; W3 "Width of wheel link (cm):"; W "Width of entire link (cm):"; T "Thickness (cm):"; Rb "Radius of base (cm):"; Ob "Base arc offset (cm):"; Rev "Reverse Bracket and Socket axes"; Lb "Supporting bracket length (cm):"; Rsh "Supporting bracket hole radius (cm):"; Rs "Wheel hub socket radius (cm):"; Hi "Wheel hub socket inner height (cm):"; Rh "Wheel hub ball radius (cm):"; Oh "Wheel hub socket offset (cm):"; rho "Density (kg/m^3):"; clr "Color ([r g b]):"
      mask help: This block models a wishbone link. The wishbone links are attached to the frame and they carry the wheel assembly. The ports A and B correspond to the frames at the hinge points where the wishbone link attaches to the chassis. The port W corresponds to the point where the wishbone link attaches to the steering knuckle.
      mask init:
      | wishbone_xsec = [Rb 0; W/2 0; W/2 L1; W/2-W3 L1; 
      |                  W/2-W3 L1-L3; -W/2 L2; -W/2 0; -Rb 0];
      | 
      | theta = linspace(pi,0,100)';
      | wishbone_xsec = [wishbone_xsec; Rb*cos(theta) Rb*sin(theta)+Ob];
      | 
      | wishbone_xsec = simmechanics.demohelpers.round_corners(wishbone_xsec, ...
      |                               [3 4 5 6], ...
      |                               [1 1 1 3], ...
      |                               5);
      | 
      | theta = linspace(3*pi/2,-pi/2,100)';
      | wishbone_xsec = [wishbone_xsec; 
      |                  wishbone_xsec(1,:);
      |                  W/2-W3/2+Rs*cos(theta) Rs*sin(theta)+L1-Oh];
      | 
      | bracket_xsec = [T/2 0; T/2 Lb; -T/2 Lb; -T/2 0];
      | bracket_xsec = simmechanics.demohelpers.round_corners(bracket_xsec,[2 3],1,5);
      | bracket_xsec = [bracket_xsec; 
      |                 bracket_xsec(1,:);
      |                 Rsh*cos(theta) Rsh*sin(theta)+Lb/2];
      mask DialogControl ParameterTabVar0 Prompt: Wishbone
      mask DialogControl ParameterTabVar01 Prompt: Brackets
      mask DialogControl ParameterTabVar012 Prompt: Socket
      mask DialogControl ParameterTabVar0123 Prompt: Material Properties
      mask Display:
      | image(imread(fullfile(matlabroot,...
      |     'toolbox','physmod','sm','smdemos',...
      |     'suspension_templates','images','sm_isuspension_wbone.png')));
      | 
      | port_label('LConn',1,'A');
      | port_label('LConn',2,'B');
      | port_label('RConn',1,'W');

== system sm_suspension_templates_lib/Double Bracket ==
  A XForm : sm_lib/Frames and Transforms/Rigid Transform  TranslationMethod=StandardAxis  TranslationStandardOffset=S/2+T/2  TranslationLengthUnit=cm  TranslationStandardAxis=+Z  TranslationCartesianOffset=[0 0 0]  TranslationROffset=0  TranslationROffsetUnits=m  TranslationZOffset=0  TranslationZOffsetUnits=m  TranslationThetaOffset=0  TranslationThetaOffsetUnits=deg  RotationMethod=None  RotationAngleUnits=deg  RotationStandardAxis=+Z  RotationAngle=0  RotationArbitraryAxis=[0 0 1]  FollAlignAxisA=+Z  BaseAlignAxisA=+Y  FollAlignAxisB=+X  BaseAlignAxisB=+X  RotationSequenceAxes=FollowerAxes  RotationSequence=XYX  RotationSequenceAngles=[0 0 0]  RotationSequenceAnglesUnits=deg  RotationMatrix=[1 0 0; 0 1 0; 0 0 1]
  B XForm : sm_lib/Frames and Transforms/Rigid Transform  TranslationMethod=StandardAxis  TranslationStandardOffset=S/2+T/2  TranslationLengthUnit=cm  TranslationStandardAxis=-Z  TranslationCartesianOffset=[0 0 0]  TranslationROffset=0  TranslationROffsetUnits=m  TranslationZOffset=0  TranslationZOffsetUnits=m  TranslationThetaOffset=0  TranslationThetaOffsetUnits=deg  RotationMethod=None  RotationAngleUnits=deg  RotationStandardAxis=+Z  RotationAngle=0  RotationArbitraryAxis=[0 0 1]  FollAlignAxisA=+Z  BaseAlignAxisA=+Y  FollAlignAxisB=+X  BaseAlignAxisB=+X  RotationSequenceAxes=FollowerAxes  RotationSequence=XYX  RotationSequenceAngles=[0 0 0]  RotationSequenceAnglesUnits=deg  RotationMatrix=[1 0 0; 0 1 0; 0 0 1]
  Base XForm : sm_lib/Frames and Transforms/Rigid Transform  TranslationMethod=StandardAxis  TranslationStandardOffset=L/2  TranslationLengthUnit=cm  TranslationStandardAxis=-Y  TranslationCartesianOffset=[0 0 0]  TranslationROffset=0  TranslationROffsetUnits=m  TranslationZOffset=0  TranslationZOffsetUnits=m  TranslationThetaOffset=0  TranslationThetaOffsetUnits=deg  RotationMethod=AlignedAxes  RotationAngleUnits=deg  RotationStandardAxis=+Z  RotationAngle=0  RotationArbitraryAxis=[0 0 1]  FollAlignAxisA=+Z  BaseAlignAxisA=+Y  FollAlignAxisB=+X  BaseAlignAxisB=+X  RotationSequenceAxes=FollowerAxes  RotationSequence=XYX  RotationSequenceAngles=[0 0 0]  RotationSequenceAnglesUnits=deg  RotationMatrix=[1 0 0; 0 1 0; 0 0 1]
  Flange A : sm_lib/Body Elements/Extruded Solid  GraphicAmbientColor=[0.15 0.15 0.15 1.0]  BasedOnType=Density  CenterOfMass=[0 0 0]  CenterOfMassUnits=m  GraphicDiffuseColor=clr  ExportConvexHullGeometry=off  ExtrusionCrossSection=bracket_xsec  ExtrusionCrossSectionUnits=cm  Density=rho  DensityUnits=kg/(m^3)  DoExposeReferenceFrame=on  GraphicEmissiveColor=[0.0 0.0 0.0 1.0]  ExportEntireGeometry=off  ExtrusionLength=T  ExtrusionLengthUnits=cm  ExtrusionType=General  SerializedFrames=<Frames/>  MarkerShape=Sphere  MarkerSize=10  GraphicType=FromGeometry  InertiaType=CalculateFromGeometry  Mass=1  MassUnits=kg  MomentsOfInertia=[1 1 1]  MomentsOfInertiaUnits=kg*m^2  PolygonNumSides=3  GraphicOpacity=1.0  PolygonOuterRadius=1  PolygonOuterRadiusUnits=m  ProductsOfInertia=[0 0 0]  ProductsOfInertiaUnits=kg*m^2  GraphicShininess=75  GraphicSpecularColor=[0.5 0.5 0.5 1.0]  GraphicVisPropType=SimpleVisualProperties
  Flange B : sm_lib/Body Elements/Extruded Solid  GraphicAmbientColor=[0.15 0.15 0.15 1.0]  BasedOnType=Density  CenterOfMass=[0 0 0]  CenterOfMassUnits=m  GraphicDiffuseColor=clr  ExportConvexHullGeometry=off  ExtrusionCrossSection=bracket_xsec  ExtrusionCrossSectionUnits=cm  Density=rho  DensityUnits=kg/(m^3)  DoExposeReferenceFrame=on  GraphicEmissiveColor=[0.0 0.0 0.0 1.0]  ExportEntireGeometry=off  ExtrusionLength=T  ExtrusionLengthUnits=cm  ExtrusionType=General  SerializedFrames=<Frames/>  MarkerShape=Sphere  MarkerSize=10  GraphicType=FromGeometry  InertiaType=CalculateFromGeometry  Mass=1  MassUnits=kg  MomentsOfInertia=[1 1 1]  MomentsOfInertiaUnits=kg*m^2  PolygonNumSides=3  GraphicOpacity=1.0  PolygonOuterRadius=1  PolygonOuterRadiusUnits=m  ProductsOfInertia=[0 0 0]  ProductsOfInertiaUnits=kg*m^2  GraphicShininess=75  GraphicSpecularColor=[0.5 0.5 0.5 1.0]  GraphicVisPropType=SimpleVisualProperties
  B : PMIOPort  Side=Right
  H : PMIOPort  Port=2  Side=Left
  connections:
  A XForm/LConn1 -- H/RConn1 -- Base XForm/LConn1 -- B XForm/LConn1
  Base XForm/RConn1 -- B/RConn1
  A XForm/RConn1 -- Flange A/RConn1
  B XForm/RConn1 -- Flange B/RConn1

== system sm_suspension_templates_lib/Forked Steering Arm ==
  Base XForm : sm_lib/Frames and Transforms/Rigid Transform  TranslationMethod=StandardAxis  TranslationStandardOffset=L-Lf+T/2  TranslationLengthUnit=cm  TranslationStandardAxis=-X  TranslationCartesianOffset=[0 0 0]  TranslationROffset=0  TranslationROffsetUnits=m  TranslationZOffset=0  TranslationZOffsetUnits=m  TranslationThetaOffset=0  TranslationThetaOffsetUnits=deg  RotationMethod=None  RotationAngleUnits=deg  RotationStandardAxis=+Z  RotationAngle=0  RotationArbitraryAxis=[0 0 1]  FollAlignAxisA=+Z  BaseAlignAxisA=-Y  FollAlignAxisB=+Y  BaseAlignAxisB=+Z  RotationSequenceAxes=FollowerAxes  RotationSequence=XYX  RotationSequenceAngles=[0 0 0]  RotationSequenceAnglesUnits=deg  RotationMatrix=[1 0 0; 0 1 0; 0 0 1]
  Forked Link : sm_lib/Body Elements/Extruded Solid  GraphicAmbientColor=[0.15 0.15 0.15 1.0]  BasedOnType=Density  CenterOfMass=[0 0 0]  CenterOfMassUnits=m  GraphicDiffuseColor=clr  ExportConvexHullGeometry=off  ExtrusionCrossSection=fork_xsec  ExtrusionCrossSectionUnits=cm  Density=rho  DensityUnits=kg/(m^3)  DoExposeReferenceFrame=on  GraphicEmissiveColor=[0.0 0.0 0.0 1.0]  ExportEntireGeometry=off  ExtrusionLength=W  ExtrusionLengthUnits=cm  ExtrusionType=General  SerializedFrames=<Frames/>  MarkerShape=Sphere  MarkerSize=10  GraphicType=FromGeometry  InertiaType=CalculateFromGeometry  Mass=1  MassUnits=kg  MomentsOfInertia=[1 1 1]  MomentsOfInertiaUnits=kg*m^2  PolygonNumSides=3  GraphicOpacity=1.0  PolygonOuterRadius=1  PolygonOuterRadiusUnits=m  ProductsOfInertia=[0 0 0]  ProductsOfInertiaUnits=kg*m^2  GraphicShininess=75  GraphicSpecularColor=[0.5 0.5 0.5 1.0]  GraphicVisPropType=SimpleVisualProperties
  Pin : sm_lib/Body Elements/Cylindrical Solid  GraphicAmbientColor=[0.15 0.15 0.15 1.0]  BasedOnType=Density  CenterOfMass=[0 0 0]  CenterOfMassUnits=m  GraphicDiffuseColor=clr  CylinderLength=Hf-2*T  CylinderLengthUnits=cm  CylinderRadius=Rp  CylinderRadiusUnits=cm  Density=rho  DensityUnits=kg/(m^3)  DoExposeReferenceFrame=on  GraphicEmissiveColor=[0.0 0.0 0.0 1.0]  ExportEntireGeometry=off  SerializedFrames=<Frames/>  MarkerShape=Sphere  MarkerSize=10  GraphicType=FromGeometry  InertiaType=CalculateFromGeometry  Mass=1  MassUnits=kg  MomentsOfInertia=[1 1 1]  MomentsOfInertiaUnits=kg*m^2  GraphicOpacity=1.0  ProductsOfInertia=[0 0 0]  ProductsOfInertiaUnits=kg*m^2  GraphicShininess=75  GraphicSpecularColor=[0.5 0.5 0.5 1.0]  GraphicVisPropType=SimpleVisualProperties
  Pin XForm : sm_lib/Frames and Transforms/Rigid Transform  TranslationMethod=Cartesian  TranslationStandardOffset=0  TranslationLengthUnit=cm  TranslationStandardAxis=+X  TranslationCartesianOffset=[(Lf+T)/2 Of 0]  TranslationROffset=0  TranslationROffsetUnits=m  TranslationZOffset=0  TranslationZOffsetUnits=m  TranslationThetaOffset=0  TranslationThetaOffsetUnits=deg  RotationMethod=AlignedAxes  RotationAngleUnits=deg  RotationStandardAxis=+Z  RotationAngle=0  RotationArbitraryAxis=[0 0 1]  FollAlignAxisA=+Z  BaseAlignAxisA=+Y  FollAlignAxisB=+Y  BaseAlignAxisB=-Z  RotationSequenceAxes=FollowerAxes  RotationSequence=XYX  RotationSequenceAngles=[0 0 0]  RotationSequenceAnglesUnits=deg  RotationMatrix=[1 0 0; 0 1 0; 0 0 1]
  B : PMIOPort  Side=Left
  P : PMIOPort  Port=2  Side=Right
  connections:
  Pin XForm/LConn1 -- Forked Link/RConn1 -- Base XForm/LConn1
  P/RConn1 -- Pin XForm/RConn1 -- Pin/RConn1
  Base XForm/RConn1 -- B/RConn1
